simulink library "constantBasisParameters_varGeom_cl"  (R2020a)
settings: Solver=VariableStepAuto  StartTime=0.0  StopTime=10.0  RelTol=1e-3
undefined symbols (not defined in the file or in its folder): HILVLCONTROLLER, hiLvlCtrl, initializeBussesFromBlock
libraries: MantaFSController_cl x1, pathFollowingControllerManta_cl x1
settings Model: Creator=mcobb  LastModifiedBy=andre
settings DataIOCC: ReturnWorkspaceOutputs=off
settings DebuggingCC: ArithmeticOperatorsInVariantConditions=warning
settings SFSimCC: CustomCodeUndefinedFunction=UseInterfaceOnly

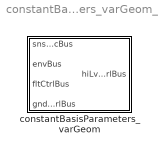
== system constantBasisParameters_varGeom_cl ==
  constantBasisParameters_varGeom : Subsystem  LoadFcn=initializeBussesFromBlock(gcb)  InitFcn=initializeBussesFromBlock(gcb)  StartFcn=initializeBussesFromBlock(gcb)  VariantControl=strcmpi(HILVLCONTROLLER,'constantBasisParameters')  mask{hiLvlCtrl=hiLvlCtrl}
      mask prompts: hiLvlCtrl "Hi-level controller"

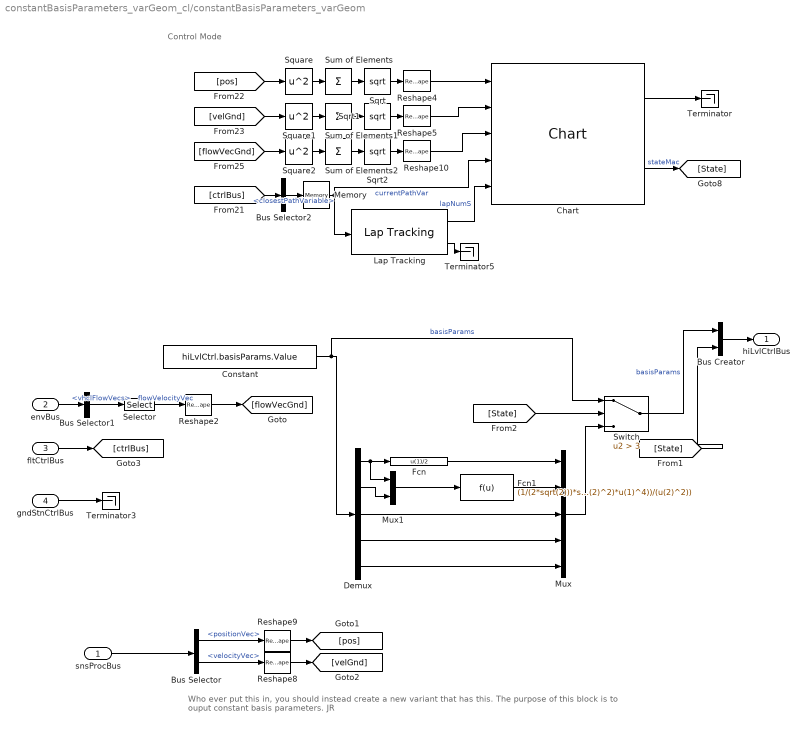
== system constantBasisParameters_varGeom_cl/constantBasisParameters_varGeom ==
  note: Who ever put this in, you should instead create a new variant that has this. The purpose of this block is to ouput constant basis parameters. JR
  note: Control Mode
  snsProcBus : Inport  OutDataTypeStr=Bus: sensorsProcessingBus
  envBus : Inport  Port=2  OutDataTypeStr=Bus: envBus
  fltCtrlBus : Inport  Port=3  OutDataTypeStr=Bus: fltCtrlBus
  gndStnCtrlBus : Inport  Port=4  OutDataTypeStr=Bus: gndStnCtrlBus
  Bus Creator : BusCreator  Inputs=2  OutDataTypeStr=Bus: hiLvlCtrlBus
  Bus Selector : BusSelector  OutputSignals=positionVec,velocityVec
  Bus Selector1 : BusSelector  OutputSignals=vhclFlowVecs
  Bus Selector2 : BusSelector  OutputSignals=closestPathVariable
  Chart : MantaFSController_cl/MantaFSController/Chart  nonXGain=fltCtrl.nonXCurrentSpoolInGain.Value  maxR=fltCtrl.maxTL.Value
  Constant : Constant  Value=hiLvlCtrl.basisParams.Value
  Demux : Demux  Outputs=5
  Fcn : Fcn  Expr=u(1)/2
  Fcn1 : Fcn  Expr=(1/(2*sqrt(2)))*sqrt(-u(1)^2+sqrt((u(2)^2*(4+u(2)^2)*u(1)^4))/(u(2)^2))
  Lap Tracking : pathFollowingControllerManta_cl/pathFollowingControllerManta/Lap Tracking  SystemSampleTime=-1  Latency=0  AutoFrameSizeCalculation=off
  Memory : Memory
  Mux : Mux  Inputs=5
  Mux1 : Mux  Inputs=2
  Reshape10 : Reshape
  Reshape2 : Reshape  OutputDimensionality=Column vector (2-D)
  Reshape4 : Reshape
  Reshape5 : Reshape
  Reshape8 : Reshape  OutputDimensionality=Column vector (2-D)
  Reshape9 : Reshape  OutputDimensionality=Column vector (2-D)
  Selector : Selector  NumberOfDimensions=2  InputPortWidth=3  IndexOptions=Select all,Index vector (dialog)  Indices=[1 3],5  OutputSizes=1,1
  Sqrt : Sqrt  SaturateOnIntegerOverflow=on
  Sqrt1 : Sqrt  SaturateOnIntegerOverflow=on
  Sqrt2 : Sqrt  SaturateOnIntegerOverflow=on
  Square : Math  Operator=square  SaturateOnIntegerOverflow=on
  Square1 : Math  Operator=square  SaturateOnIntegerOverflow=on
  Square2 : Math  Operator=square  SaturateOnIntegerOverflow=on
  Sum of Elements : Sum  Inputs=+
  Sum of Elements1 : Sum  Inputs=+
  Sum of Elements2 : Sum  Inputs=+
  Switch : Switch  Criteria=u2 > Threshold  Threshold=3
  Terminator : Terminator
  Terminator3 : Terminator
  Terminator5 : Terminator
  hiLvlCtrlBus : Outport  OutDataTypeStr=Bus: hiLvlCtrlBus  VectorParamsAs1DForOutWhenUnconnected=off
  wires:
  gndStnCtrlBus/1 -> Terminator3/1
  Bus Creator/1 -> hiLvlCtrlBus/1
  fltCtrlBus/1 -> [ctrlBus]
  Constant/1 -> Switch/1, Demux/1  "basisParams"
  Demux/5 -> Mux/5
  Demux/4 -> Mux/4
  Demux/3 -> Mux/3
  Demux/1 -> Mux1/1, Fcn/1
  Fcn/1 -> Mux/1
  Demux/2 -> Mux1/2
  Mux1/1 -> Fcn1/1
  Fcn1/1 -> Mux/2
  Mux/1 -> Switch/3
  Switch/1 -> Bus Creator/1  "basisParams"
  [State] -> Switch/2
  Square2/1 -> Sum of Elements2/1
  [velGnd] -> Square1/1
  [flowVecGnd] -> Square2/1
  Square/1 -> Sum of Elements/1
  Sqrt1/1 -> Reshape5/1
  Sum of Elements/1 -> Sqrt/1
  Reshape5/1 -> Chart/2
  Chart/1 -> Terminator/1
  [ctrlBus] -> Bus Selector2/1
  Chart/2 -> [State]  "stateMac"
  Bus Selector2/1 -> Memory/1  "<closestPathVariable>"
  Lap Tracking/1 -> Chart/5  "lapNumS"
  Reshape4/1 -> Chart/1
  Sqrt/1 -> Reshape4/1
  Square1/1 -> Sum of Elements1/1
  Memory/1 -> Lap Tracking/1, Chart/4  "currentPathVar"
  Lap Tracking/2 -> Terminator5/1
  Reshape10/1 -> Chart/3
  [pos] -> Square/1
  Sum of Elements2/1 -> Sqrt2/1
  Sqrt2/1 -> Reshape10/1
  Sum of Elements1/1 -> Sqrt1/1
  Reshape9/1 -> [pos]
  snsProcBus/1 -> Bus Selector/1
  Reshape8/1 -> [velGnd]
  Bus Selector/2 -> Reshape8/1  "<velocityVec>"
  Bus Selector/1 -> Reshape9/1  "<positionVec>"
  Bus Selector1/1 -> Selector/1  "<vhclFlowVecs>"
  Reshape2/1 -> [flowVecGnd]
  envBus/1 -> Bus Selector1/1
  Selector/1 -> Reshape2/1  "flowVelocityVec"
  [State] -> Bus Creator/2
